simulink model "Katex_FullCar_R2017b_V03"  (R2026a)
settings: Solver=ode1  StopTime=1000  FixedStep=Ts  EnableMultiTasking=on
PostLoadFcn:
  | , if any(exist('dsrtsu_mdlpostloadfcn', 'file') == [2, 3, 6]), try dsrtsu_mdlpostloadfcn('Execute', bdroot); catch fprintf('Error in PostLoadFcn (dsrtsu_mdlpostloadfcn) for model "%s":\n %s\n', bdroot, lasterr); end, end,
  | , if any(exist('dsrtsu_mdlpostloadfcn', 'file') ~= 0), dsrtsu_mdlpostloadfcn('Execute', bdroot); end,
InitFcn:
  | , if any(exist('rtifpga_mdlclblib', 'file') ~= 0), rtifpga_mdlclblib('Init', bdroot); end,
  | 
  | 
  | init
undefined symbols (not defined in the file): locklim_sus, roundN, Ts
libraries: sl_discontinuities x29, simulink_extras x26, simulink x22, mjLib x1
(part 8 of 10)

== system Katex_FullCar_R2017b_V03/DGIST/_Low_Level_Ctrl/Steering_Low_Level_Controller/Torque Mode/Steering Motor Control/Lag compensator(zeta)/a//(s+p) ==
  note: y(n) = [(2-p*Ts)*y(n-1)+a*Ts(u(n)+u(n-1))]/(2+p*Ts)
  note: H(s) = a/(s+p)
  note: s = 2/Ts*(z-1)/(z+1)
  In : Inport
  a : Inport  Port=2
  p : Inport  Port=3
  Constant : Constant  Value=2  SampleTime=Ts
  Product1 : Product  Inputs=*/  RndMeth=Zero
  Product11 : Product  RndMeth=Zero
  Product3 : Product  RndMeth=Zero
  Sum1 : Sum  Inputs=-+  InputSameDT=on  SaturateOnIntegerOverflow=on  OutDataTypeStr=Inherit: Same as first input
  Sum2 : Sum  InputSameDT=on  SaturateOnIntegerOverflow=on  OutDataTypeStr=Inherit: Same as first input
  Sum3 : Sum  InputSameDT=on  SaturateOnIntegerOverflow=on  OutDataTypeStr=Inherit: Same as first input
  Sum4 : Sum  InputSameDT=on  SaturateOnIntegerOverflow=on  OutDataTypeStr=Inherit: Same as first input
  d : UnitDelay  SampleTime=Ts
  d1 : UnitDelay  SampleTime=Ts
  gain : Gain  Gain=Ts  SaturateOnIntegerOverflow=on  OutDataTypeStr=Inherit: Same as input  ParamDataTypeStr=Inherit: Same as input
  gain1 : Gain  Gain=Ts  SaturateOnIntegerOverflow=on  OutDataTypeStr=Inherit: Same as input  ParamDataTypeStr=Inherit: Same as input
  Out : Outport  VectorParamsAs1DForOutWhenUnconnected=off
  wires:
  In/1 -> Sum3/1, d1/1
  d1/1 -> Sum3/2
  Sum3/1 -> gain/1
  Product11/1 -> Sum2/2
  Sum1/1 -> Product11/1
  Constant/1 -> Sum1/2, Sum4/2
  p/1 -> gain1/1
  gain1/1 -> Sum1/1, Sum4/1
  d/1 -> Product11/2
  Sum2/1 -> Product1/1
  Sum4/1 -> Product1/2
  Product1/1 -> Out/1, d/1
  gain/1 -> Product3/1
  a/1 -> Product3/2
  Product3/1 -> Sum2/1

== system Katex_FullCar_R2017b_V03/DGIST/_Low_Level_Ctrl/Steering_Low_Level_Controller/Torque Mode/Steering Motor Control/Poleplacement(PI)1/Integrator1 ==
  note: Integrator
  in : Inport
  "Off : 0 On : 1" : Inport  Port=2
  Divide : Product  Inputs=**
  Sum1 : Sum  InputSameDT=on  SaturateOnIntegerOverflow=on  OutDataTypeStr=Inherit: Same as first input
  Sum2 : Sum  InputSameDT=on  SaturateOnIntegerOverflow=on  OutDataTypeStr=Inherit: Same as first input
  d : UnitDelay  SampleTime=Ts
  d1 : UnitDelay  SampleTime=Ts
  gain : Gain  Gain=Ts/2  SaturateOnIntegerOverflow=on  OutDataTypeStr=Inherit: Same as input  ParamDataTypeStr=Inherit: Same as input
  out : Outport  VectorParamsAs1DForOutWhenUnconnected=off
  wires:
  gain/1 -> Sum2/1
  Sum1/1 -> gain/1
  d1/1 -> Sum1/2
  in/1 -> d1/1, Sum1/1
  Sum2/1 -> Divide/1, out/1
  d/1 -> Sum2/2
  Divide/1 -> d/1
  "Off : 0 On : 1"/1 -> Divide/2

== system Katex_FullCar_R2017b_V03/DGIST/_Low_Level_Ctrl/Steering_Low_Level_Controller/Torque Mode/Steering Motor Control/Steering Ref Mode /If Action Subsystem ==
  In1 : Inport
  Action Port : ActionPort
  Out1 : Outport  VectorParamsAs1DForOutWhenUnconnected=off
  wires:
  In1/1 -> Out1/1

== system Katex_FullCar_R2017b_V03/DGIST/_Low_Level_Ctrl/Steering_Low_Level_Controller/Torque Mode/Steering Motor Control/Steering Ref Mode /If Action Subsystem1 ==
  In1 : Inport
  Action Port : ActionPort
  Out1 : Outport  VectorParamsAs1DForOutWhenUnconnected=off
  wires:
  In1/1 -> Out1/1

== system Katex_FullCar_R2017b_V03/DGIST/_Low_Level_Ctrl/Steering_Low_Level_Controller/Torque Mode/Steering Motor Control/Steering Ref Mode /If Action Subsystem2 ==
  In1 : Inport
  Action Port : ActionPort
  Out1 : Outport  VectorParamsAs1DForOutWhenUnconnected=off
  wires:
  In1/1 -> Out1/1

== system Katex_FullCar_R2017b_V03/DGIST/_Low_Level_Ctrl/Steering_Low_Level_Controller/Torque Mode/Steering Motor Control1/DOB(theta)/Dot ==
  note: Dot
  in : Inport
  Sum1 : Sum  Inputs=+-  InputSameDT=on  SaturateOnIntegerOverflow=on  OutDataTypeStr=Inherit: Same as first input
  Sum2 : Sum  Inputs=+-  InputSameDT=on  SaturateOnIntegerOverflow=on  OutDataTypeStr=Inherit: Same as first input
  d : UnitDelay  SampleTime=Ts
  d1 : UnitDelay  SampleTime=Ts
  gain : Gain  Gain=2/Ts  SaturateOnIntegerOverflow=on  OutDataTypeStr=Inherit: Same as input  ParamDataTypeStr=Inherit: Same as input
  out : Outport  VectorParamsAs1DForOutWhenUnconnected=off
  wires:
  Sum1/1 -> d1/1, out/1
  d1/1 -> Sum1/2
  Sum2/1 -> gain/1
  in/1 -> d/1, Sum2/1
  d/1 -> Sum2/2
  gain/1 -> Sum1/1

== system Katex_FullCar_R2017b_V03/DGIST/_Low_Level_Ctrl/Steering_Low_Level_Controller/Torque Mode/Steering Motor Control1/DOB(theta)/Dot1 ==
  note: Dot
  in : Inport
  Sum1 : Sum  Inputs=+-  InputSameDT=on  SaturateOnIntegerOverflow=on  OutDataTypeStr=Inherit: Same as first input
  Sum2 : Sum  Inputs=+-  InputSameDT=on  SaturateOnIntegerOverflow=on  OutDataTypeStr=Inherit: Same as first input
  d : UnitDelay  SampleTime=Ts
  d1 : UnitDelay  SampleTime=Ts
  gain : Gain  Gain=2/Ts  SaturateOnIntegerOverflow=on  OutDataTypeStr=Inherit: Same as input  ParamDataTypeStr=Inherit: Same as input
  out : Outport  VectorParamsAs1DForOutWhenUnconnected=off
  wires:
  Sum1/1 -> d1/1, out/1
  d1/1 -> Sum1/2
  Sum2/1 -> gain/1
  in/1 -> d/1, Sum2/1
  d/1 -> Sum2/2
  gain/1 -> Sum1/1

== system Katex_FullCar_R2017b_V03/DGIST/_Low_Level_Ctrl/Steering_Low_Level_Controller/Torque Mode/Steering Motor Control1/DOB(theta)/Dot2 ==
  note: Dot
  in : Inport
  Sum1 : Sum  Inputs=+-  InputSameDT=on  SaturateOnIntegerOverflow=on  OutDataTypeStr=Inherit: Same as first input
  Sum2 : Sum  Inputs=+-  InputSameDT=on  SaturateOnIntegerOverflow=on  OutDataTypeStr=Inherit: Same as first input
  d : UnitDelay  SampleTime=Ts
  d1 : UnitDelay  SampleTime=Ts
  gain : Gain  Gain=2/Ts  SaturateOnIntegerOverflow=on  OutDataTypeStr=Inherit: Same as input  ParamDataTypeStr=Inherit: Same as input
  out : Outport  VectorParamsAs1DForOutWhenUnconnected=off
  wires:
  Sum1/1 -> d1/1, out/1
  d1/1 -> Sum1/2
  Sum2/1 -> gain/1
  in/1 -> d/1, Sum2/1
  d/1 -> Sum2/2
  gain/1 -> Sum1/1

== system Katex_FullCar_R2017b_V03/DGIST/_Low_Level_Ctrl/Steering_Low_Level_Controller/Torque Mode/Steering Motor Control1/DOB(theta)/Second order LPF ==
  note: y(n) = [Ts^2*w^2*{x(n)+2*x(n-1)+x(n-2)}-(2*w^2*Ts^2-8)*y(n-1)-(4+w^2*Ts^2+2*zeta*Ts*w)*y(n-2)]
      | /(4+w^2*Ts^2+2*zeta*Ts*w)
  note: H(s) = w^2/(s^2+2*zeta*w*s+w^2)
  note: s = 2/Ts*(z-1)/(z+1)
  In : Inport
  fc : Inport  Port=2
  zeta : Inport  Port=3
  Constant : Constant  Value=Ts  SampleTime=Ts
  Constant1 : Constant  Value=8  SampleTime=Ts
  Constant2 : Constant  Value=4  SampleTime=Ts
  Delay : Delay  InitialCondition=0  SampleTime=Ts
  Delay1 : Delay  DelayLength=1  InitialCondition=0  SampleTime=Ts
  Delay2 : Delay  DelayLength=1  InitialCondition=0  SampleTime=Ts
  Delay3 : Delay  InitialCondition=0  SampleTime=Ts
  Product1 : Product  Inputs=*/  RndMeth=Zero
  Product2 : Product  Inputs=4  RndMeth=Zero
  Product3 : Product  RndMeth=Zero
  Product4 : Product  RndMeth=Zero
  Sum1 : Sum  Inputs=+-  InputSameDT=on  SaturateOnIntegerOverflow=on  OutDataTypeStr=Inherit: Same as first input
  Sum2 : Sum  Inputs=+-  InputSameDT=on  SaturateOnIntegerOverflow=on  OutDataTypeStr=Inherit: Same as first input
  Sum3 : Sum  Inputs=+++  InputSameDT=on  SaturateOnIntegerOverflow=on  OutDataTypeStr=Inherit: Same as first input
  Sum4 : Sum  Inputs=+-  InputSameDT=on  SaturateOnIntegerOverflow=on  OutDataTypeStr=Inherit: Same as first input
  Sum5 : Sum  Inputs=+-+  InputSameDT=on  SaturateOnIntegerOverflow=on  OutDataTypeStr=Inherit: Same as first input
  Sum6 : Sum  Inputs=+++  InputSameDT=on  SaturateOnIntegerOverflow=on  OutDataTypeStr=Inherit: Same as first input
  gain1 : Gain  Gain=2  SaturateOnIntegerOverflow=on  OutDataTypeStr=Inherit: Same as input  ParamDataTypeStr=Inherit: Same as input
  gain2 : Gain  Gain=2*pi  SaturateOnIntegerOverflow=on  OutDataTypeStr=Inherit: Same as input  ParamDataTypeStr=Inherit: Same as input
  gain3 : Gain  Gain=2  SaturateOnIntegerOverflow=on  OutDataTypeStr=Inherit: Same as input  ParamDataTypeStr=Inherit: Same as input
  gain4 : Gain  Gain=4  SaturateOnIntegerOverflow=on  OutDataTypeStr=Inherit: Same as input  ParamDataTypeStr=Inherit: Same as input
  "x(n), x(n-1), x(n-2)" : Product  RndMeth=Zero
  y(n-1) : Product  RndMeth=Zero
  y(n-2) : Product  RndMeth=Zero
  Dist_hat : Outport  VectorParamsAs1DForOutWhenUnconnected=off
  wires:
  Product1/1 -> Dist_hat/1, Delay3/1, Delay2/1
  Sum2/1 -> Product1/1
  fc/1 -> gain2/1
  In/1 -> Delay1/1, Delay/1, Sum3/1
  gain2/1 -> Product3/1, Product2/2, Product2/1
  Constant/1 -> Product3/2, Product2/4, Product2/3
  Delay1/1 -> gain1/1
  gain1/1 -> Sum3/2
  Delay/1 -> Sum3/3
  Sum3/1 -> "x(n), x(n-1), x(n-2)"/1
  Product2/1 -> Sum5/1, Sum6/1, "x(n), x(n-1), x(n-2)"/2, gain3/1
  "x(n), x(n-1), x(n-2)"/1 -> Sum1/1
  Sum1/1 -> Sum2/1
  y(n-1)/1 -> Sum1/2
  Sum4/1 -> y(n-1)/1
  gain3/1 -> Sum4/1
  Constant1/1 -> Sum4/2
  Delay2/1 -> y(n-1)/2
  Product3/1 -> gain4/1
  Constant2/1 -> Sum5/3, Sum6/3
  Sum5/1 -> y(n-2)/1
  Delay3/1 -> y(n-2)/2
  y(n-2)/1 -> Sum2/2
  Sum6/1 -> Product1/2
  zeta/1 -> Product4/2
  gain4/1 -> Product4/1
  Product4/1 -> Sum6/2, Sum5/2

== system Katex_FullCar_R2017b_V03/DGIST/_Low_Level_Ctrl/Steering_Low_Level_Controller/Torque Mode/Steering Motor Control1/Feedforward(theta)/Dot ==
  note: Dot
  in : Inport
  Sum1 : Sum  Inputs=+-  InputSameDT=on  SaturateOnIntegerOverflow=on  OutDataTypeStr=Inherit: Same as first input
  Sum2 : Sum  Inputs=+-  InputSameDT=on  SaturateOnIntegerOverflow=on  OutDataTypeStr=Inherit: Same as first input
  d : UnitDelay  SampleTime=Ts
  d1 : UnitDelay  SampleTime=Ts
  gain : Gain  Gain=2/Ts  SaturateOnIntegerOverflow=on  OutDataTypeStr=Inherit: Same as input  ParamDataTypeStr=Inherit: Same as input
  out : Outport  VectorParamsAs1DForOutWhenUnconnected=off
  wires:
  Sum1/1 -> d1/1, out/1
  d1/1 -> Sum1/2
  Sum2/1 -> gain/1
  in/1 -> d/1, Sum2/1
  d/1 -> Sum2/2
  gain/1 -> Sum1/1

== system Katex_FullCar_R2017b_V03/DGIST/_Low_Level_Ctrl/Steering_Low_Level_Controller/Torque Mode/Steering Motor Control1/Feedforward(theta)/Dot1 ==
  note: Dot
  in : Inport
  Sum1 : Sum  Inputs=+-  InputSameDT=on  SaturateOnIntegerOverflow=on  OutDataTypeStr=Inherit: Same as first input
  Sum2 : Sum  Inputs=+-  InputSameDT=on  SaturateOnIntegerOverflow=on  OutDataTypeStr=Inherit: Same as first input
  d : UnitDelay  SampleTime=Ts
  d1 : UnitDelay  SampleTime=Ts
  gain : Gain  Gain=2/Ts  SaturateOnIntegerOverflow=on  OutDataTypeStr=Inherit: Same as input  ParamDataTypeStr=Inherit: Same as input
  out : Outport  VectorParamsAs1DForOutWhenUnconnected=off
  wires:
  Sum1/1 -> d1/1, out/1
  d1/1 -> Sum1/2
  Sum2/1 -> gain/1
  in/1 -> d/1, Sum2/1
  d/1 -> Sum2/2
  gain/1 -> Sum1/1

== system Katex_FullCar_R2017b_V03/DGIST/_Low_Level_Ctrl/Steering_Low_Level_Controller/Torque Mode/Steering Motor Control1/Feedforward(theta)/Dot2 ==
  note: Dot
  in : Inport
  Sum1 : Sum  Inputs=+-  InputSameDT=on  SaturateOnIntegerOverflow=on  OutDataTypeStr=Inherit: Same as first input
  Sum2 : Sum  Inputs=+-  InputSameDT=on  SaturateOnIntegerOverflow=on  OutDataTypeStr=Inherit: Same as first input
  d : UnitDelay  SampleTime=Ts
  d1 : UnitDelay  SampleTime=Ts
  gain : Gain  Gain=2/Ts  SaturateOnIntegerOverflow=on  OutDataTypeStr=Inherit: Same as input  ParamDataTypeStr=Inherit: Same as input
  out : Outport  VectorParamsAs1DForOutWhenUnconnected=off
  wires:
  Sum1/1 -> d1/1, out/1
  d1/1 -> Sum1/2
  Sum2/1 -> gain/1
  in/1 -> d/1, Sum2/1
  d/1 -> Sum2/2
  gain/1 -> Sum1/1

== system Katex_FullCar_R2017b_V03/DGIST/_Low_Level_Ctrl/Steering_Low_Level_Controller/Torque Mode/Steering Motor Control1/Feedforward(theta)/Second order LPF ==
  note: y(n) = [Ts^2*w^2*{x(n)+2*x(n-1)+x(n-2)}-(2*w^2*Ts^2-8)*y(n-1)-(4+w^2*Ts^2+2*zeta*Ts*w)*y(n-2)]
      | /(4+w^2*Ts^2+2*zeta*Ts*w)
  note: H(s) = w^2/(s^2+2*zeta*w*s+w^2)
  note: s = 2/Ts*(z-1)/(z+1)
  In : Inport
  fc : Inport  Port=2
  zeta : Inport  Port=3
  Constant : Constant  Value=Ts  SampleTime=Ts
  Constant1 : Constant  Value=8  SampleTime=Ts
  Constant2 : Constant  Value=4  SampleTime=Ts
  Delay : Delay  InitialCondition=0  SampleTime=Ts
  Delay1 : Delay  DelayLength=1  InitialCondition=0  SampleTime=Ts
  Delay2 : Delay  DelayLength=1  InitialCondition=0  SampleTime=Ts
  Delay3 : Delay  InitialCondition=0  SampleTime=Ts
  Product1 : Product  Inputs=*/  RndMeth=Zero
  Product2 : Product  Inputs=4  RndMeth=Zero
  Product3 : Product  RndMeth=Zero
  Product4 : Product  RndMeth=Zero
  Sum1 : Sum  Inputs=+-  InputSameDT=on  SaturateOnIntegerOverflow=on  OutDataTypeStr=Inherit: Same as first input
  Sum2 : Sum  Inputs=+-  InputSameDT=on  SaturateOnIntegerOverflow=on  OutDataTypeStr=Inherit: Same as first input
  Sum3 : Sum  Inputs=+++  InputSameDT=on  SaturateOnIntegerOverflow=on  OutDataTypeStr=Inherit: Same as first input
  Sum4 : Sum  Inputs=+-  InputSameDT=on  SaturateOnIntegerOverflow=on  OutDataTypeStr=Inherit: Same as first input
  Sum5 : Sum  Inputs=+-+  InputSameDT=on  SaturateOnIntegerOverflow=on  OutDataTypeStr=Inherit: Same as first input
  Sum6 : Sum  Inputs=+++  InputSameDT=on  SaturateOnIntegerOverflow=on  OutDataTypeStr=Inherit: Same as first input
  gain1 : Gain  Gain=2  SaturateOnIntegerOverflow=on  OutDataTypeStr=Inherit: Same as input  ParamDataTypeStr=Inherit: Same as input
  gain2 : Gain  Gain=2*pi  SaturateOnIntegerOverflow=on  OutDataTypeStr=Inherit: Same as input  ParamDataTypeStr=Inherit: Same as input
  gain3 : Gain  Gain=2  SaturateOnIntegerOverflow=on  OutDataTypeStr=Inherit: Same as input  ParamDataTypeStr=Inherit: Same as input
  gain4 : Gain  Gain=4  SaturateOnIntegerOverflow=on  OutDataTypeStr=Inherit: Same as input  ParamDataTypeStr=Inherit: Same as input
  "x(n), x(n-1), x(n-2)" : Product  RndMeth=Zero
  y(n-1) : Product  RndMeth=Zero
  y(n-2) : Product  RndMeth=Zero
  Out : Outport  VectorParamsAs1DForOutWhenUnconnected=off
  wires:
  Product1/1 -> Out/1, Delay3/1, Delay2/1
  Sum2/1 -> Product1/1
  fc/1 -> gain2/1
  In/1 -> Delay1/1, Delay/1, Sum3/1
  gain2/1 -> Product3/1, Product2/2, Product2/1
  Constant/1 -> Product3/2, Product2/4, Product2/3
  Delay1/1 -> gain1/1
  gain1/1 -> Sum3/2
  Delay/1 -> Sum3/3
  Sum3/1 -> "x(n), x(n-1), x(n-2)"/1
  Product2/1 -> Sum5/1, Sum6/1, "x(n), x(n-1), x(n-2)"/2, gain3/1
  "x(n), x(n-1), x(n-2)"/1 -> Sum1/1
  Sum1/1 -> Sum2/1
  y(n-1)/1 -> Sum1/2
  Sum4/1 -> y(n-1)/1
  gain3/1 -> Sum4/1
  Constant1/1 -> Sum4/2
  Delay2/1 -> y(n-1)/2
  Product3/1 -> gain4/1
  Constant2/1 -> Sum5/3, Sum6/3
  Sum5/1 -> y(n-2)/1
  Delay3/1 -> y(n-2)/2
  y(n-2)/1 -> Sum2/2
  Sum6/1 -> Product1/2
  zeta/1 -> Product4/2
  gain4/1 -> Product4/1
  Product4/1 -> Sum6/2, Sum5/2

== system Katex_FullCar_R2017b_V03/DGIST/_Low_Level_Ctrl/Steering_Low_Level_Controller/Torque Mode/Steering Motor Control1/Lag compensator(zeta)/Dot1 ==
  note: Dot
  in : Inport
  Sum1 : Sum  Inputs=+-  InputSameDT=on  SaturateOnIntegerOverflow=on  OutDataTypeStr=Inherit: Same as first input
  Sum2 : Sum  Inputs=+-  InputSameDT=on  SaturateOnIntegerOverflow=on  OutDataTypeStr=Inherit: Same as first input
  d : UnitDelay  SampleTime=Ts
  d1 : UnitDelay  SampleTime=Ts
  gain : Gain  Gain=2/Ts  SaturateOnIntegerOverflow=on  OutDataTypeStr=Inherit: Same as input  ParamDataTypeStr=Inherit: Same as input
  out : Outport  VectorParamsAs1DForOutWhenUnconnected=off
  wires:
  Sum1/1 -> d1/1, out/1
  d1/1 -> Sum1/2
  Sum2/1 -> gain/1
  in/1 -> d/1, Sum2/1
  d/1 -> Sum2/2
  gain/1 -> Sum1/1

== system Katex_FullCar_R2017b_V03/DGIST/_Low_Level_Ctrl/Steering_Low_Level_Controller/Torque Mode/Steering Motor Control1/Lag compensator(zeta)/a//(s+p) ==
  note: y(n) = [(2-p*Ts)*y(n-1)+a*Ts(u(n)+u(n-1))]/(2+p*Ts)
  note: H(s) = a/(s+p)
  note: s = 2/Ts*(z-1)/(z+1)
  In : Inport
  a : Inport  Port=2
  p : Inport  Port=3
  Constant : Constant  Value=2  SampleTime=Ts
  Product1 : Product  Inputs=*/  RndMeth=Zero
  Product11 : Product  RndMeth=Zero
  Product3 : Product  RndMeth=Zero
  Sum1 : Sum  Inputs=-+  InputSameDT=on  SaturateOnIntegerOverflow=on  OutDataTypeStr=Inherit: Same as first input
  Sum2 : Sum  InputSameDT=on  SaturateOnIntegerOverflow=on  OutDataTypeStr=Inherit: Same as first input
  Sum3 : Sum  InputSameDT=on  SaturateOnIntegerOverflow=on  OutDataTypeStr=Inherit: Same as first input
  Sum4 : Sum  InputSameDT=on  SaturateOnIntegerOverflow=on  OutDataTypeStr=Inherit: Same as first input
  d : UnitDelay  SampleTime=Ts
  d1 : UnitDelay  SampleTime=Ts
  gain : Gain  Gain=Ts  SaturateOnIntegerOverflow=on  OutDataTypeStr=Inherit: Same as input  ParamDataTypeStr=Inherit: Same as input
  gain1 : Gain  Gain=Ts  SaturateOnIntegerOverflow=on  OutDataTypeStr=Inherit: Same as input  ParamDataTypeStr=Inherit: Same as input
  Out : Outport  VectorParamsAs1DForOutWhenUnconnected=off
  wires:
  In/1 -> Sum3/1, d1/1
  d1/1 -> Sum3/2
  Sum3/1 -> gain/1
  Product11/1 -> Sum2/2
  Sum1/1 -> Product11/1
  Constant/1 -> Sum1/2, Sum4/2
  p/1 -> gain1/1
  gain1/1 -> Sum1/1, Sum4/1
  d/1 -> Product11/2
  Sum2/1 -> Product1/1
  Sum4/1 -> Product1/2
  Product1/1 -> Out/1, d/1
  gain/1 -> Product3/1
  a/1 -> Product3/2
  Product3/1 -> Sum2/1

== system Katex_FullCar_R2017b_V03/DGIST/_Low_Level_Ctrl/Steering_Low_Level_Controller/Torque Mode/Steering Motor Control2/DOB(omega)/Dot2 ==
  note: Dot
  in : Inport
  Sum1 : Sum  Inputs=+-  InputSameDT=on  SaturateOnIntegerOverflow=on  OutDataTypeStr=Inherit: Same as first input
  Sum2 : Sum  Inputs=+-  InputSameDT=on  SaturateOnIntegerOverflow=on  OutDataTypeStr=Inherit: Same as first input
  d : UnitDelay  SampleTime=Ts
  d1 : UnitDelay  SampleTime=Ts
  gain : Gain  Gain=2/Ts  SaturateOnIntegerOverflow=on  OutDataTypeStr=Inherit: Same as input  ParamDataTypeStr=Inherit: Same as input
  out : Outport  VectorParamsAs1DForOutWhenUnconnected=off
  wires:
  Sum1/1 -> d1/1, out/1
  d1/1 -> Sum1/2
  Sum2/1 -> gain/1
  in/1 -> d/1, Sum2/1
  d/1 -> Sum2/2
  gain/1 -> Sum1/1

== system Katex_FullCar_R2017b_V03/DGIST/_Low_Level_Ctrl/Steering_Low_Level_Controller/Torque Mode/Steering Motor Control2/DOB(omega)/LPF ==
  note: LPF : tau = 1/(2*pi*fc)
  note: y(n) = [Ts*{x(n)+x(n-1)}+(2*tau-Ts)*y(n-1)]/(2*tau+Ts)
  note: H(s) = 1/(tau*s+1)
  note: s = 2/Ts*(z-1)/(z+1)
  In : Inport
  fc : Inport  Port=2
  Constant : Constant  Value=Ts  SampleTime=Ts
  Constant1 : Constant  SampleTime=Ts
  Product1 : Product  Inputs=*/  RndMeth=Zero
  Product11 : Product  RndMeth=Zero
  Product2 : Product  Inputs=*/  RndMeth=Zero
  Sum1 : Sum  Inputs=+-  InputSameDT=on  SaturateOnIntegerOverflow=on  OutDataTypeStr=Inherit: Same as first input
  Sum2 : Sum  InputSameDT=on  SaturateOnIntegerOverflow=on  OutDataTypeStr=Inherit: Same as first input
  Sum3 : Sum  InputSameDT=on  SaturateOnIntegerOverflow=on  OutDataTypeStr=Inherit: Same as first input
  Sum4 : Sum  InputSameDT=on  SaturateOnIntegerOverflow=on  OutDataTypeStr=Inherit: Same as first input
  d : UnitDelay  SampleTime=Ts
  d1 : UnitDelay  SampleTime=Ts
  gain : Gain  Gain=Ts  SaturateOnIntegerOverflow=on  OutDataTypeStr=Inherit: Same as input  ParamDataTypeStr=Inherit: Same as input
  gain1 : Gain  Gain=2  SaturateOnIntegerOverflow=on  OutDataTypeStr=Inherit: Same as input  ParamDataTypeStr=Inherit: Same as input
  gain2 : Gain  Gain=2*pi  SaturateOnIntegerOverflow=on  OutDataTypeStr=Inherit: Same as input  ParamDataTypeStr=Inherit: Same as input
  Out : Outport  VectorParamsAs1DForOutWhenUnconnected=off
  wires:
  In/1 -> Sum3/1, d1/1
  d1/1 -> Sum3/2
  Sum3/1 -> gain/1
  gain/1 -> Sum2/1
  Product11/1 -> Sum2/2
  Sum1/1 -> Product11/1
  Constant/1 -> Sum1/2, Sum4/2
  fc/1 -> gain2/1
  gain1/1 -> Sum1/1, Sum4/1
  d/1 -> Product11/2
  Sum2/1 -> Product1/1
  Sum4/1 -> Product1/2
  Product1/1 -> Out/1, d/1
  Product2/1 -> gain1/1
  Constant1/1 -> Product2/1
  gain2/1 -> Product2/2

== system Katex_FullCar_R2017b_V03/DGIST/_Low_Level_Ctrl/Steering_Low_Level_Controller/Torque Mode/Steering Motor Control2/DOB(theta)/Dot ==
  note: Dot
  in : Inport
  Sum1 : Sum  Inputs=+-  InputSameDT=on  SaturateOnIntegerOverflow=on  OutDataTypeStr=Inherit: Same as first input
  Sum2 : Sum  Inputs=+-  InputSameDT=on  SaturateOnIntegerOverflow=on  OutDataTypeStr=Inherit: Same as first input
  d : UnitDelay  SampleTime=Ts
  d1 : UnitDelay  SampleTime=Ts
  gain : Gain  Gain=2/Ts  SaturateOnIntegerOverflow=on  OutDataTypeStr=Inherit: Same as input  ParamDataTypeStr=Inherit: Same as input
  out : Outport  VectorParamsAs1DForOutWhenUnconnected=off
  wires:
  Sum1/1 -> d1/1, out/1
  d1/1 -> Sum1/2
  Sum2/1 -> gain/1
  in/1 -> d/1, Sum2/1
  d/1 -> Sum2/2
  gain/1 -> Sum1/1

== system Katex_FullCar_R2017b_V03/DGIST/_Low_Level_Ctrl/Steering_Low_Level_Controller/Torque Mode/Steering Motor Control2/DOB(theta)/Dot1 ==
  note: Dot
  in : Inport
  Sum1 : Sum  Inputs=+-  InputSameDT=on  SaturateOnIntegerOverflow=on  OutDataTypeStr=Inherit: Same as first input
  Sum2 : Sum  Inputs=+-  InputSameDT=on  SaturateOnIntegerOverflow=on  OutDataTypeStr=Inherit: Same as first input
  d : UnitDelay  SampleTime=Ts
  d1 : UnitDelay  SampleTime=Ts
  gain : Gain  Gain=2/Ts  SaturateOnIntegerOverflow=on  OutDataTypeStr=Inherit: Same as input  ParamDataTypeStr=Inherit: Same as input
  out : Outport  VectorParamsAs1DForOutWhenUnconnected=off
  wires:
  Sum1/1 -> d1/1, out/1
  d1/1 -> Sum1/2
  Sum2/1 -> gain/1
  in/1 -> d/1, Sum2/1
  d/1 -> Sum2/2
  gain/1 -> Sum1/1

== system Katex_FullCar_R2017b_V03/DGIST/_Low_Level_Ctrl/Steering_Low_Level_Controller/Torque Mode/Steering Motor Control2/DOB(theta)/Dot2 ==
  note: Dot
  in : Inport
  Sum1 : Sum  Inputs=+-  InputSameDT=on  SaturateOnIntegerOverflow=on  OutDataTypeStr=Inherit: Same as first input
  Sum2 : Sum  Inputs=+-  InputSameDT=on  SaturateOnIntegerOverflow=on  OutDataTypeStr=Inherit: Same as first input
  d : UnitDelay  SampleTime=Ts
  d1 : UnitDelay  SampleTime=Ts
  gain : Gain  Gain=2/Ts  SaturateOnIntegerOverflow=on  OutDataTypeStr=Inherit: Same as input  ParamDataTypeStr=Inherit: Same as input
  out : Outport  VectorParamsAs1DForOutWhenUnconnected=off
  wires:
  Sum1/1 -> d1/1, out/1
  d1/1 -> Sum1/2
  Sum2/1 -> gain/1
  in/1 -> d/1, Sum2/1
  d/1 -> Sum2/2
  gain/1 -> Sum1/1

== system Katex_FullCar_R2017b_V03/DGIST/_Low_Level_Ctrl/Steering_Low_Level_Controller/Torque Mode/Steering Motor Control2/DOB(theta)/Second order LPF ==
  note: y(n) = [Ts^2*w^2*{x(n)+2*x(n-1)+x(n-2)}-(2*w^2*Ts^2-8)*y(n-1)-(4+w^2*Ts^2+2*zeta*Ts*w)*y(n-2)]
      | /(4+w^2*Ts^2+2*zeta*Ts*w)
  note: H(s) = w^2/(s^2+2*zeta*w*s+w^2)
  note: s = 2/Ts*(z-1)/(z+1)
  In : Inport
  fc : Inport  Port=2
  zeta : Inport  Port=3
  Constant : Constant  Value=Ts  SampleTime=Ts
  Constant1 : Constant  Value=8  SampleTime=Ts
  Constant2 : Constant  Value=4  SampleTime=Ts
  Delay : Delay  InitialCondition=0  SampleTime=Ts
  Delay1 : Delay  DelayLength=1  InitialCondition=0  SampleTime=Ts
  Delay2 : Delay  DelayLength=1  InitialCondition=0  SampleTime=Ts
  Delay3 : Delay  InitialCondition=0  SampleTime=Ts
  Product1 : Product  Inputs=*/  RndMeth=Zero
  Product2 : Product  Inputs=4  RndMeth=Zero
  Product3 : Product  RndMeth=Zero
  Product4 : Product  RndMeth=Zero
  Sum1 : Sum  Inputs=+-  InputSameDT=on  SaturateOnIntegerOverflow=on  OutDataTypeStr=Inherit: Same as first input
  Sum2 : Sum  Inputs=+-  InputSameDT=on  SaturateOnIntegerOverflow=on  OutDataTypeStr=Inherit: Same as first input
  Sum3 : Sum  Inputs=+++  InputSameDT=on  SaturateOnIntegerOverflow=on  OutDataTypeStr=Inherit: Same as first input
  Sum4 : Sum  Inputs=+-  InputSameDT=on  SaturateOnIntegerOverflow=on  OutDataTypeStr=Inherit: Same as first input
  Sum5 : Sum  Inputs=+-+  InputSameDT=on  SaturateOnIntegerOverflow=on  OutDataTypeStr=Inherit: Same as first input
  Sum6 : Sum  Inputs=+++  InputSameDT=on  SaturateOnIntegerOverflow=on  OutDataTypeStr=Inherit: Same as first input
  gain1 : Gain  Gain=2  SaturateOnIntegerOverflow=on  OutDataTypeStr=Inherit: Same as input  ParamDataTypeStr=Inherit: Same as input
  gain2 : Gain  Gain=2*pi  SaturateOnIntegerOverflow=on  OutDataTypeStr=Inherit: Same as input  ParamDataTypeStr=Inherit: Same as input
  gain3 : Gain  Gain=2  SaturateOnIntegerOverflow=on  OutDataTypeStr=Inherit: Same as input  ParamDataTypeStr=Inherit: Same as input
  gain4 : Gain  Gain=4  SaturateOnIntegerOverflow=on  OutDataTypeStr=Inherit: Same as input  ParamDataTypeStr=Inherit: Same as input
  "x(n), x(n-1), x(n-2)" : Product  RndMeth=Zero
  y(n-1) : Product  RndMeth=Zero
  y(n-2) : Product  RndMeth=Zero
  Dist_hat : Outport  VectorParamsAs1DForOutWhenUnconnected=off
  wires:
  Product1/1 -> Dist_hat/1, Delay3/1, Delay2/1
  Sum2/1 -> Product1/1
  fc/1 -> gain2/1
  In/1 -> Delay1/1, Delay/1, Sum3/1
  gain2/1 -> Product3/1, Product2/2, Product2/1
  Constant/1 -> Product3/2, Product2/4, Product2/3
  Delay1/1 -> gain1/1
  gain1/1 -> Sum3/2
  Delay/1 -> Sum3/3
  Sum3/1 -> "x(n), x(n-1), x(n-2)"/1
  Product2/1 -> Sum5/1, Sum6/1, "x(n), x(n-1), x(n-2)"/2, gain3/1
  "x(n), x(n-1), x(n-2)"/1 -> Sum1/1
  Sum1/1 -> Sum2/1
  y(n-1)/1 -> Sum1/2
  Sum4/1 -> y(n-1)/1
  gain3/1 -> Sum4/1
  Constant1/1 -> Sum4/2
  Delay2/1 -> y(n-1)/2
  Product3/1 -> gain4/1
  Constant2/1 -> Sum5/3, Sum6/3
  Sum5/1 -> y(n-2)/1
  Delay3/1 -> y(n-2)/2
  y(n-2)/1 -> Sum2/2
  Sum6/1 -> Product1/2
  zeta/1 -> Product4/2
  gain4/1 -> Product4/1
  Product4/1 -> Sum6/2, Sum5/2

== system Katex_FullCar_R2017b_V03/DGIST/_Low_Level_Ctrl/Steering_Low_Level_Controller/Torque Mode/Steering Motor Control2/Feedforward(omega)/Dot2 ==
  note: Dot
  in : Inport
  Sum1 : Sum  Inputs=+-  InputSameDT=on  SaturateOnIntegerOverflow=on  OutDataTypeStr=Inherit: Same as first input
  Sum2 : Sum  Inputs=+-  InputSameDT=on  SaturateOnIntegerOverflow=on  OutDataTypeStr=Inherit: Same as first input
  d : UnitDelay  SampleTime=Ts
  d1 : UnitDelay  SampleTime=Ts
  gain : Gain  Gain=2/Ts  SaturateOnIntegerOverflow=on  OutDataTypeStr=Inherit: Same as input  ParamDataTypeStr=Inherit: Same as input
  out : Outport  VectorParamsAs1DForOutWhenUnconnected=off
  wires:
  Sum1/1 -> d1/1, out/1
  d1/1 -> Sum1/2
  Sum2/1 -> gain/1
  in/1 -> d/1, Sum2/1
  d/1 -> Sum2/2
  gain/1 -> Sum1/1

== system Katex_FullCar_R2017b_V03/DGIST/_Low_Level_Ctrl/Steering_Low_Level_Controller/Torque Mode/Steering Motor Control2/Feedforward(omega)/LPF ==
  note: LPF : tau = 1/(2*pi*fc)
  note: y(n) = [Ts*{x(n)+x(n-1)}+(2*tau-Ts)*y(n-1)]/(2*tau+Ts)
  note: H(s) = 1/(tau*s+1)
  note: s = 2/Ts*(z-1)/(z+1)
  In : Inport
  fc : Inport  Port=2
  Constant : Constant  Value=Ts  SampleTime=Ts
  Constant1 : Constant  SampleTime=Ts
  Product1 : Product  Inputs=*/  RndMeth=Zero
  Product11 : Product  RndMeth=Zero
  Product2 : Product  Inputs=*/  RndMeth=Zero
  Sum1 : Sum  Inputs=+-  InputSameDT=on  SaturateOnIntegerOverflow=on  OutDataTypeStr=Inherit: Same as first input
  Sum2 : Sum  InputSameDT=on  SaturateOnIntegerOverflow=on  OutDataTypeStr=Inherit: Same as first input
  Sum3 : Sum  InputSameDT=on  SaturateOnIntegerOverflow=on  OutDataTypeStr=Inherit: Same as first input
  Sum4 : Sum  InputSameDT=on  SaturateOnIntegerOverflow=on  OutDataTypeStr=Inherit: Same as first input
  d : UnitDelay  SampleTime=Ts
  d1 : UnitDelay  SampleTime=Ts
  gain : Gain  Gain=Ts  SaturateOnIntegerOverflow=on  OutDataTypeStr=Inherit: Same as input  ParamDataTypeStr=Inherit: Same as input
  gain1 : Gain  Gain=2  SaturateOnIntegerOverflow=on  OutDataTypeStr=Inherit: Same as input  ParamDataTypeStr=Inherit: Same as input
  gain2 : Gain  Gain=2*pi  SaturateOnIntegerOverflow=on  OutDataTypeStr=Inherit: Same as input  ParamDataTypeStr=Inherit: Same as input
  Out : Outport  VectorParamsAs1DForOutWhenUnconnected=off
  wires:
  In/1 -> Sum3/1, d1/1
  d1/1 -> Sum3/2
  Sum3/1 -> gain/1
  gain/1 -> Sum2/1
  Product11/1 -> Sum2/2
  Sum1/1 -> Product11/1
  Constant/1 -> Sum1/2, Sum4/2
  fc/1 -> gain2/1
  gain1/1 -> Sum1/1, Sum4/1
  d/1 -> Product11/2
  Sum2/1 -> Product1/1
  Sum4/1 -> Product1/2
  Product1/1 -> Out/1, d/1
  Product2/1 -> gain1/1
  Constant1/1 -> Product2/1
  gain2/1 -> Product2/2

== system Katex_FullCar_R2017b_V03/DGIST/_Low_Level_Ctrl/Steering_Low_Level_Controller/Torque Mode/Steering Motor Control2/Feedforward(theta)/Dot ==
  note: Dot
  in : Inport
  Sum1 : Sum  Inputs=+-  InputSameDT=on  SaturateOnIntegerOverflow=on  OutDataTypeStr=Inherit: Same as first input
  Sum2 : Sum  Inputs=+-  InputSameDT=on  SaturateOnIntegerOverflow=on  OutDataTypeStr=Inherit: Same as first input
  d : UnitDelay  SampleTime=Ts
  d1 : UnitDelay  SampleTime=Ts
  gain : Gain  Gain=2/Ts  SaturateOnIntegerOverflow=on  OutDataTypeStr=Inherit: Same as input  ParamDataTypeStr=Inherit: Same as input
  out : Outport  VectorParamsAs1DForOutWhenUnconnected=off
  wires:
  Sum1/1 -> d1/1, out/1
  d1/1 -> Sum1/2
  Sum2/1 -> gain/1
  in/1 -> d/1, Sum2/1
  d/1 -> Sum2/2
  gain/1 -> Sum1/1

== system Katex_FullCar_R2017b_V03/DGIST/_Low_Level_Ctrl/Steering_Low_Level_Controller/Torque Mode/Steering Motor Control2/Feedforward(theta)/Dot1 ==
  note: Dot
  in : Inport
  Sum1 : Sum  Inputs=+-  InputSameDT=on  SaturateOnIntegerOverflow=on  OutDataTypeStr=Inherit: Same as first input
  Sum2 : Sum  Inputs=+-  InputSameDT=on  SaturateOnIntegerOverflow=on  OutDataTypeStr=Inherit: Same as first input
  d : UnitDelay  SampleTime=Ts
  d1 : UnitDelay  SampleTime=Ts
  gain : Gain  Gain=2/Ts  SaturateOnIntegerOverflow=on  OutDataTypeStr=Inherit: Same as input  ParamDataTypeStr=Inherit: Same as input
  out : Outport  VectorParamsAs1DForOutWhenUnconnected=off
  wires:
  Sum1/1 -> d1/1, out/1
  d1/1 -> Sum1/2
  Sum2/1 -> gain/1
  in/1 -> d/1, Sum2/1
  d/1 -> Sum2/2
  gain/1 -> Sum1/1

== system Katex_FullCar_R2017b_V03/DGIST/_Low_Level_Ctrl/Steering_Low_Level_Controller/Torque Mode/Steering Motor Control2/Feedforward(theta)/Dot2 ==
  note: Dot
  in : Inport
  Sum1 : Sum  Inputs=+-  InputSameDT=on  SaturateOnIntegerOverflow=on  OutDataTypeStr=Inherit: Same as first input
  Sum2 : Sum  Inputs=+-  InputSameDT=on  SaturateOnIntegerOverflow=on  OutDataTypeStr=Inherit: Same as first input
  d : UnitDelay  SampleTime=Ts
  d1 : UnitDelay  SampleTime=Ts
  gain : Gain  Gain=2/Ts  SaturateOnIntegerOverflow=on  OutDataTypeStr=Inherit: Same as input  ParamDataTypeStr=Inherit: Same as input
  out : Outport  VectorParamsAs1DForOutWhenUnconnected=off
  wires:
  Sum1/1 -> d1/1, out/1
  d1/1 -> Sum1/2
  Sum2/1 -> gain/1
  in/1 -> d/1, Sum2/1
  d/1 -> Sum2/2
  gain/1 -> Sum1/1

== system Katex_FullCar_R2017b_V03/DGIST/_Low_Level_Ctrl/Steering_Low_Level_Controller/Torque Mode/Steering Motor Control2/Feedforward(theta)/Second order LPF ==
  note: y(n) = [Ts^2*w^2*{x(n)+2*x(n-1)+x(n-2)}-(2*w^2*Ts^2-8)*y(n-1)-(4+w^2*Ts^2+2*zeta*Ts*w)*y(n-2)]
      | /(4+w^2*Ts^2+2*zeta*Ts*w)
  note: H(s) = w^2/(s^2+2*zeta*w*s+w^2)
  note: s = 2/Ts*(z-1)/(z+1)
  In : Inport
  fc : Inport  Port=2
  zeta : Inport  Port=3
  Constant : Constant  Value=Ts  SampleTime=Ts
  Constant1 : Constant  Value=8  SampleTime=Ts
  Constant2 : Constant  Value=4  SampleTime=Ts
  Delay : Delay  InitialCondition=0  SampleTime=Ts
  Delay1 : Delay  DelayLength=1  InitialCondition=0  SampleTime=Ts
  Delay2 : Delay  DelayLength=1  InitialCondition=0  SampleTime=Ts
  Delay3 : Delay  InitialCondition=0  SampleTime=Ts
  Product1 : Product  Inputs=*/  RndMeth=Zero
  Product2 : Product  Inputs=4  RndMeth=Zero
  Product3 : Product  RndMeth=Zero
  Product4 : Product  RndMeth=Zero
  Sum1 : Sum  Inputs=+-  InputSameDT=on  SaturateOnIntegerOverflow=on  OutDataTypeStr=Inherit: Same as first input
  Sum2 : Sum  Inputs=+-  InputSameDT=on  SaturateOnIntegerOverflow=on  OutDataTypeStr=Inherit: Same as first input
  Sum3 : Sum  Inputs=+++  InputSameDT=on  SaturateOnIntegerOverflow=on  OutDataTypeStr=Inherit: Same as first input
  Sum4 : Sum  Inputs=+-  InputSameDT=on  SaturateOnIntegerOverflow=on  OutDataTypeStr=Inherit: Same as first input
  Sum5 : Sum  Inputs=+-+  InputSameDT=on  SaturateOnIntegerOverflow=on  OutDataTypeStr=Inherit: Same as first input
  Sum6 : Sum  Inputs=+++  InputSameDT=on  SaturateOnIntegerOverflow=on  OutDataTypeStr=Inherit: Same as first input
  gain1 : Gain  Gain=2  SaturateOnIntegerOverflow=on  OutDataTypeStr=Inherit: Same as input  ParamDataTypeStr=Inherit: Same as input
  gain2 : Gain  Gain=2*pi  SaturateOnIntegerOverflow=on  OutDataTypeStr=Inherit: Same as input  ParamDataTypeStr=Inherit: Same as input
  gain3 : Gain  Gain=2  SaturateOnIntegerOverflow=on  OutDataTypeStr=Inherit: Same as input  ParamDataTypeStr=Inherit: Same as input
  gain4 : Gain  Gain=4  SaturateOnIntegerOverflow=on  OutDataTypeStr=Inherit: Same as input  ParamDataTypeStr=Inherit: Same as input
  "x(n), x(n-1), x(n-2)" : Product  RndMeth=Zero
  y(n-1) : Product  RndMeth=Zero
  y(n-2) : Product  RndMeth=Zero
  Out : Outport  VectorParamsAs1DForOutWhenUnconnected=off
  wires:
  Product1/1 -> Out/1, Delay3/1, Delay2/1
  Sum2/1 -> Product1/1
  fc/1 -> gain2/1
  In/1 -> Delay1/1, Delay/1, Sum3/1
  gain2/1 -> Product3/1, Product2/2, Product2/1
  Constant/1 -> Product3/2, Product2/4, Product2/3
  Delay1/1 -> gain1/1
  gain1/1 -> Sum3/2
  Delay/1 -> Sum3/3
  Sum3/1 -> "x(n), x(n-1), x(n-2)"/1
  Product2/1 -> Sum5/1, Sum6/1, "x(n), x(n-1), x(n-2)"/2, gain3/1
  "x(n), x(n-1), x(n-2)"/1 -> Sum1/1
  Sum1/1 -> Sum2/1
  y(n-1)/1 -> Sum1/2
  Sum4/1 -> y(n-1)/1
  gain3/1 -> Sum4/1
  Constant1/1 -> Sum4/2
  Delay2/1 -> y(n-1)/2
  Product3/1 -> gain4/1
  Constant2/1 -> Sum5/3, Sum6/3
  Sum5/1 -> y(n-2)/1
  Delay3/1 -> y(n-2)/2
  y(n-2)/1 -> Sum2/2
  Sum6/1 -> Product1/2
  zeta/1 -> Product4/2
  gain4/1 -> Product4/1
  Product4/1 -> Sum6/2, Sum5/2

== system Katex_FullCar_R2017b_V03/DGIST/_Low_Level_Ctrl/Steering_Low_Level_Controller/Torque Mode/Steering Motor Control2/Lag compensator(zeta)/Dot1 ==
  note: Dot
  in : Inport
  Sum1 : Sum  Inputs=+-  InputSameDT=on  SaturateOnIntegerOverflow=on  OutDataTypeStr=Inherit: Same as first input
  Sum2 : Sum  Inputs=+-  InputSameDT=on  SaturateOnIntegerOverflow=on  OutDataTypeStr=Inherit: Same as first input
  d : UnitDelay  SampleTime=Ts
  d1 : UnitDelay  SampleTime=Ts
  gain : Gain  Gain=2/Ts  SaturateOnIntegerOverflow=on  OutDataTypeStr=Inherit: Same as input  ParamDataTypeStr=Inherit: Same as input
  out : Outport  VectorParamsAs1DForOutWhenUnconnected=off
  wires:
  Sum1/1 -> d1/1, out/1
  d1/1 -> Sum1/2
  Sum2/1 -> gain/1
  in/1 -> d/1, Sum2/1
  d/1 -> Sum2/2
  gain/1 -> Sum1/1

== system Katex_FullCar_R2017b_V03/DGIST/_Low_Level_Ctrl/Steering_Low_Level_Controller/Torque Mode/Steering Motor Control2/Lag compensator(zeta)/a//(s+p) ==
  note: y(n) = [(2-p*Ts)*y(n-1)+a*Ts(u(n)+u(n-1))]/(2+p*Ts)
  note: H(s) = a/(s+p)
  note: s = 2/Ts*(z-1)/(z+1)
  In : Inport
  a : Inport  Port=2
  p : Inport  Port=3
  Constant : Constant  Value=2  SampleTime=Ts
  Product1 : Product  Inputs=*/  RndMeth=Zero
  Product11 : Product  RndMeth=Zero
  Product3 : Product  RndMeth=Zero
  Sum1 : Sum  Inputs=-+  InputSameDT=on  SaturateOnIntegerOverflow=on  OutDataTypeStr=Inherit: Same as first input
  Sum2 : Sum  InputSameDT=on  SaturateOnIntegerOverflow=on  OutDataTypeStr=Inherit: Same as first input
  Sum3 : Sum  InputSameDT=on  SaturateOnIntegerOverflow=on  OutDataTypeStr=Inherit: Same as first input
  Sum4 : Sum  InputSameDT=on  SaturateOnIntegerOverflow=on  OutDataTypeStr=Inherit: Same as first input
  d : UnitDelay  SampleTime=Ts
  d1 : UnitDelay  SampleTime=Ts
  gain : Gain  Gain=Ts  SaturateOnIntegerOverflow=on  OutDataTypeStr=Inherit: Same as input  ParamDataTypeStr=Inherit: Same as input
  gain1 : Gain  Gain=Ts  SaturateOnIntegerOverflow=on  OutDataTypeStr=Inherit: Same as input  ParamDataTypeStr=Inherit: Same as input
  Out : Outport  VectorParamsAs1DForOutWhenUnconnected=off
  wires:
  In/1 -> Sum3/1, d1/1
  d1/1 -> Sum3/2
  Sum3/1 -> gain/1
  Product11/1 -> Sum2/2
  Sum1/1 -> Product11/1
  Constant/1 -> Sum1/2, Sum4/2
  p/1 -> gain1/1
  gain1/1 -> Sum1/1, Sum4/1
  d/1 -> Product11/2
  Sum2/1 -> Product1/1
  Sum4/1 -> Product1/2
  Product1/1 -> Out/1, d/1
  gain/1 -> Product3/1
  a/1 -> Product3/2
  Product3/1 -> Sum2/1

== system Katex_FullCar_R2017b_V03/DGIST/_Low_Level_Ctrl/Steering_Low_Level_Controller/Torque Mode/Steering Motor Control2/Poleplacement(PI)1/Integrator1 ==
  note: Integrator
  in : Inport
  "Off : 0 On : 1" : Inport  Port=2
  Divide : Product  Inputs=**
  Sum1 : Sum  InputSameDT=on  SaturateOnIntegerOverflow=on  OutDataTypeStr=Inherit: Same as first input
  Sum2 : Sum  InputSameDT=on  SaturateOnIntegerOverflow=on  OutDataTypeStr=Inherit: Same as first input
  d : UnitDelay  SampleTime=Ts
  d1 : UnitDelay  SampleTime=Ts
  gain : Gain  Gain=Ts/2  SaturateOnIntegerOverflow=on  OutDataTypeStr=Inherit: Same as input  ParamDataTypeStr=Inherit: Same as input
  out : Outport  VectorParamsAs1DForOutWhenUnconnected=off
  wires:
  gain/1 -> Sum2/1
  Sum1/1 -> gain/1
  d1/1 -> Sum1/2
  in/1 -> d1/1, Sum1/1
  Sum2/1 -> Divide/1, out/1
  d/1 -> Sum2/2
  Divide/1 -> d/1
  "Off : 0 On : 1"/1 -> Divide/2

== system Katex_FullCar_R2017b_V03/DGIST/_Low_Level_Ctrl/Steering_Low_Level_Controller/Torque Mode/Steering Motor Control2/Steering Ref Mode /If Action Subsystem ==
  In1 : Inport
  Action Port : ActionPort
  Out1 : Outport  VectorParamsAs1DForOutWhenUnconnected=off
  wires:
  In1/1 -> Out1/1

== system Katex_FullCar_R2017b_V03/DGIST/_Low_Level_Ctrl/Steering_Low_Level_Controller/Torque Mode/Steering Motor Control2/Steering Ref Mode /If Action Subsystem1 ==
  In1 : Inport
  Action Port : ActionPort
  Out1 : Outport  VectorParamsAs1DForOutWhenUnconnected=off
  wires:
  In1/1 -> Out1/1

== system Katex_FullCar_R2017b_V03/DGIST/_Low_Level_Ctrl/Steering_Low_Level_Controller/Torque Mode/Steering Motor Control2/Steering Ref Mode /If Action Subsystem2 ==
  In1 : Inport
  Action Port : ActionPort
  Out1 : Outport  VectorParamsAs1DForOutWhenUnconnected=off
  wires:
  In1/1 -> Out1/1

== system Katex_FullCar_R2017b_V03/DGIST/_Low_Level_Ctrl/Steering_Low_Level_Controller/Torque Mode/Steering Motor Control3/DOB(theta)/Dot ==
  note: Dot
  in : Inport
  Sum1 : Sum  Inputs=+-  InputSameDT=on  SaturateOnIntegerOverflow=on  OutDataTypeStr=Inherit: Same as first input
  Sum2 : Sum  Inputs=+-  InputSameDT=on  SaturateOnIntegerOverflow=on  OutDataTypeStr=Inherit: Same as first input
  d : UnitDelay  SampleTime=Ts
  d1 : UnitDelay  SampleTime=Ts
  gain : Gain  Gain=2/Ts  SaturateOnIntegerOverflow=on  OutDataTypeStr=Inherit: Same as input  ParamDataTypeStr=Inherit: Same as input
  out : Outport  VectorParamsAs1DForOutWhenUnconnected=off
  wires:
  Sum1/1 -> d1/1, out/1
  d1/1 -> Sum1/2
  Sum2/1 -> gain/1
  in/1 -> d/1, Sum2/1
  d/1 -> Sum2/2
  gain/1 -> Sum1/1

== system Katex_FullCar_R2017b_V03/DGIST/_Low_Level_Ctrl/Steering_Low_Level_Controller/Torque Mode/Steering Motor Control3/DOB(theta)/Dot1 ==
  note: Dot
  in : Inport
  Sum1 : Sum  Inputs=+-  InputSameDT=on  SaturateOnIntegerOverflow=on  OutDataTypeStr=Inherit: Same as first input
  Sum2 : Sum  Inputs=+-  InputSameDT=on  SaturateOnIntegerOverflow=on  OutDataTypeStr=Inherit: Same as first input
  d : UnitDelay  SampleTime=Ts
  d1 : UnitDelay  SampleTime=Ts
  gain : Gain  Gain=2/Ts  SaturateOnIntegerOverflow=on  OutDataTypeStr=Inherit: Same as input  ParamDataTypeStr=Inherit: Same as input
  out : Outport  VectorParamsAs1DForOutWhenUnconnected=off
  wires:
  Sum1/1 -> d1/1, out/1
  d1/1 -> Sum1/2
  Sum2/1 -> gain/1
  in/1 -> d/1, Sum2/1
  d/1 -> Sum2/2
  gain/1 -> Sum1/1

== system Katex_FullCar_R2017b_V03/DGIST/_Low_Level_Ctrl/Steering_Low_Level_Controller/Torque Mode/Steering Motor Control3/DOB(theta)/Dot2 ==
  note: Dot
  in : Inport
  Sum1 : Sum  Inputs=+-  InputSameDT=on  SaturateOnIntegerOverflow=on  OutDataTypeStr=Inherit: Same as first input
  Sum2 : Sum  Inputs=+-  InputSameDT=on  SaturateOnIntegerOverflow=on  OutDataTypeStr=Inherit: Same as first input
  d : UnitDelay  SampleTime=Ts
  d1 : UnitDelay  SampleTime=Ts
  gain : Gain  Gain=2/Ts  SaturateOnIntegerOverflow=on  OutDataTypeStr=Inherit: Same as input  ParamDataTypeStr=Inherit: Same as input
  out : Outport  VectorParamsAs1DForOutWhenUnconnected=off
  wires:
  Sum1/1 -> d1/1, out/1
  d1/1 -> Sum1/2
  Sum2/1 -> gain/1
  in/1 -> d/1, Sum2/1
  d/1 -> Sum2/2
  gain/1 -> Sum1/1

== system Katex_FullCar_R2017b_V03/DGIST/_Low_Level_Ctrl/Steering_Low_Level_Controller/Torque Mode/Steering Motor Control3/DOB(theta)/Second order LPF ==
  note: y(n) = [Ts^2*w^2*{x(n)+2*x(n-1)+x(n-2)}-(2*w^2*Ts^2-8)*y(n-1)-(4+w^2*Ts^2+2*zeta*Ts*w)*y(n-2)]
      | /(4+w^2*Ts^2+2*zeta*Ts*w)
  note: H(s) = w^2/(s^2+2*zeta*w*s+w^2)
  note: s = 2/Ts*(z-1)/(z+1)
  In : Inport
  fc : Inport  Port=2
  zeta : Inport  Port=3
  Constant : Constant  Value=Ts  SampleTime=Ts
  Constant1 : Constant  Value=8  SampleTime=Ts
  Constant2 : Constant  Value=4  SampleTime=Ts
  Delay : Delay  InitialCondition=0  SampleTime=Ts
  Delay1 : Delay  DelayLength=1  InitialCondition=0  SampleTime=Ts
  Delay2 : Delay  DelayLength=1  InitialCondition=0  SampleTime=Ts
  Delay3 : Delay  InitialCondition=0  SampleTime=Ts
  Product1 : Product  Inputs=*/  RndMeth=Zero
  Product2 : Product  Inputs=4  RndMeth=Zero
  Product3 : Product  RndMeth=Zero
  Product4 : Product  RndMeth=Zero
  Sum1 : Sum  Inputs=+-  InputSameDT=on  SaturateOnIntegerOverflow=on  OutDataTypeStr=Inherit: Same as first input
  Sum2 : Sum  Inputs=+-  InputSameDT=on  SaturateOnIntegerOverflow=on  OutDataTypeStr=Inherit: Same as first input
  Sum3 : Sum  Inputs=+++  InputSameDT=on  SaturateOnIntegerOverflow=on  OutDataTypeStr=Inherit: Same as first input
  Sum4 : Sum  Inputs=+-  InputSameDT=on  SaturateOnIntegerOverflow=on  OutDataTypeStr=Inherit: Same as first input
  Sum5 : Sum  Inputs=+-+  InputSameDT=on  SaturateOnIntegerOverflow=on  OutDataTypeStr=Inherit: Same as first input
  Sum6 : Sum  Inputs=+++  InputSameDT=on  SaturateOnIntegerOverflow=on  OutDataTypeStr=Inherit: Same as first input
  gain1 : Gain  Gain=2  SaturateOnIntegerOverflow=on  OutDataTypeStr=Inherit: Same as input  ParamDataTypeStr=Inherit: Same as input
  gain2 : Gain  Gain=2*pi  SaturateOnIntegerOverflow=on  OutDataTypeStr=Inherit: Same as input  ParamDataTypeStr=Inherit: Same as input
  gain3 : Gain  Gain=2  SaturateOnIntegerOverflow=on  OutDataTypeStr=Inherit: Same as input  ParamDataTypeStr=Inherit: Same as input
  gain4 : Gain  Gain=4  SaturateOnIntegerOverflow=on  OutDataTypeStr=Inherit: Same as input  ParamDataTypeStr=Inherit: Same as input
  "x(n), x(n-1), x(n-2)" : Product  RndMeth=Zero
  y(n-1) : Product  RndMeth=Zero
  y(n-2) : Product  RndMeth=Zero
  Dist_hat : Outport  VectorParamsAs1DForOutWhenUnconnected=off
  wires:
  Product1/1 -> Dist_hat/1, Delay3/1, Delay2/1
  Sum2/1 -> Product1/1
  fc/1 -> gain2/1
  In/1 -> Delay1/1, Delay/1, Sum3/1
  gain2/1 -> Product3/1, Product2/2, Product2/1
  Constant/1 -> Product3/2, Product2/4, Product2/3
  Delay1/1 -> gain1/1
  gain1/1 -> Sum3/2
  Delay/1 -> Sum3/3
  Sum3/1 -> "x(n), x(n-1), x(n-2)"/1
  Product2/1 -> Sum5/1, Sum6/1, "x(n), x(n-1), x(n-2)"/2, gain3/1
  "x(n), x(n-1), x(n-2)"/1 -> Sum1/1
  Sum1/1 -> Sum2/1
  y(n-1)/1 -> Sum1/2
  Sum4/1 -> y(n-1)/1
  gain3/1 -> Sum4/1
  Constant1/1 -> Sum4/2
  Delay2/1 -> y(n-1)/2
  Product3/1 -> gain4/1
  Constant2/1 -> Sum5/3, Sum6/3
  Sum5/1 -> y(n-2)/1
  Delay3/1 -> y(n-2)/2
  y(n-2)/1 -> Sum2/2
  Sum6/1 -> Product1/2
  zeta/1 -> Product4/2
  gain4/1 -> Product4/1
  Product4/1 -> Sum6/2, Sum5/2

== system Katex_FullCar_R2017b_V03/DGIST/_Low_Level_Ctrl/Steering_Low_Level_Controller/Torque Mode/Steering Motor Control3/Feedforward(theta)/Dot ==
  note: Dot
  in : Inport
  Sum1 : Sum  Inputs=+-  InputSameDT=on  SaturateOnIntegerOverflow=on  OutDataTypeStr=Inherit: Same as first input
  Sum2 : Sum  Inputs=+-  InputSameDT=on  SaturateOnIntegerOverflow=on  OutDataTypeStr=Inherit: Same as first input
  d : UnitDelay  SampleTime=Ts
  d1 : UnitDelay  SampleTime=Ts
  gain : Gain  Gain=2/Ts  SaturateOnIntegerOverflow=on  OutDataTypeStr=Inherit: Same as input  ParamDataTypeStr=Inherit: Same as input
  out : Outport  VectorParamsAs1DForOutWhenUnconnected=off
  wires:
  Sum1/1 -> d1/1, out/1
  d1/1 -> Sum1/2
  Sum2/1 -> gain/1
  in/1 -> d/1, Sum2/1
  d/1 -> Sum2/2
  gain/1 -> Sum1/1

== system Katex_FullCar_R2017b_V03/DGIST/_Low_Level_Ctrl/Steering_Low_Level_Controller/Torque Mode/Steering Motor Control3/Feedforward(theta)/Dot1 ==
  note: Dot
  in : Inport
  Sum1 : Sum  Inputs=+-  InputSameDT=on  SaturateOnIntegerOverflow=on  OutDataTypeStr=Inherit: Same as first input
  Sum2 : Sum  Inputs=+-  InputSameDT=on  SaturateOnIntegerOverflow=on  OutDataTypeStr=Inherit: Same as first input
  d : UnitDelay  SampleTime=Ts
  d1 : UnitDelay  SampleTime=Ts
  gain : Gain  Gain=2/Ts  SaturateOnIntegerOverflow=on  OutDataTypeStr=Inherit: Same as input  ParamDataTypeStr=Inherit: Same as input
  out : Outport  VectorParamsAs1DForOutWhenUnconnected=off
  wires:
  Sum1/1 -> d1/1, out/1
  d1/1 -> Sum1/2
  Sum2/1 -> gain/1
  in/1 -> d/1, Sum2/1
  d/1 -> Sum2/2
  gain/1 -> Sum1/1

== system Katex_FullCar_R2017b_V03/DGIST/_Low_Level_Ctrl/Steering_Low_Level_Controller/Torque Mode/Steering Motor Control3/Feedforward(theta)/Dot2 ==
  note: Dot
  in : Inport
  Sum1 : Sum  Inputs=+-  InputSameDT=on  SaturateOnIntegerOverflow=on  OutDataTypeStr=Inherit: Same as first input
  Sum2 : Sum  Inputs=+-  InputSameDT=on  SaturateOnIntegerOverflow=on  OutDataTypeStr=Inherit: Same as first input
  d : UnitDelay  SampleTime=Ts
  d1 : UnitDelay  SampleTime=Ts
  gain : Gain  Gain=2/Ts  SaturateOnIntegerOverflow=on  OutDataTypeStr=Inherit: Same as input  ParamDataTypeStr=Inherit: Same as input
  out : Outport  VectorParamsAs1DForOutWhenUnconnected=off
  wires:
  Sum1/1 -> d1/1, out/1
  d1/1 -> Sum1/2
  Sum2/1 -> gain/1
  in/1 -> d/1, Sum2/1
  d/1 -> Sum2/2
  gain/1 -> Sum1/1

== system Katex_FullCar_R2017b_V03/DGIST/_Low_Level_Ctrl/Steering_Low_Level_Controller/Torque Mode/Steering Motor Control3/Feedforward(theta)/Second order LPF ==
  note: y(n) = [Ts^2*w^2*{x(n)+2*x(n-1)+x(n-2)}-(2*w^2*Ts^2-8)*y(n-1)-(4+w^2*Ts^2+2*zeta*Ts*w)*y(n-2)]
      | /(4+w^2*Ts^2+2*zeta*Ts*w)
  note: H(s) = w^2/(s^2+2*zeta*w*s+w^2)
  note: s = 2/Ts*(z-1)/(z+1)
  In : Inport
  fc : Inport  Port=2
  zeta : Inport  Port=3
  Constant : Constant  Value=Ts  SampleTime=Ts
  Constant1 : Constant  Value=8  SampleTime=Ts
  Constant2 : Constant  Value=4  SampleTime=Ts
  Delay : Delay  InitialCondition=0  SampleTime=Ts
  Delay1 : Delay  DelayLength=1  InitialCondition=0  SampleTime=Ts
  Delay2 : Delay  DelayLength=1  InitialCondition=0  SampleTime=Ts
  Delay3 : Delay  InitialCondition=0  SampleTime=Ts
  Product1 : Product  Inputs=*/  RndMeth=Zero
  Product2 : Product  Inputs=4  RndMeth=Zero
  Product3 : Product  RndMeth=Zero
  Product4 : Product  RndMeth=Zero
  Sum1 : Sum  Inputs=+-  InputSameDT=on  SaturateOnIntegerOverflow=on  OutDataTypeStr=Inherit: Same as first input
  Sum2 : Sum  Inputs=+-  InputSameDT=on  SaturateOnIntegerOverflow=on  OutDataTypeStr=Inherit: Same as first input
  Sum3 : Sum  Inputs=+++  InputSameDT=on  SaturateOnIntegerOverflow=on  OutDataTypeStr=Inherit: Same as first input
  Sum4 : Sum  Inputs=+-  InputSameDT=on  SaturateOnIntegerOverflow=on  OutDataTypeStr=Inherit: Same as first input
  Sum5 : Sum  Inputs=+-+  InputSameDT=on  SaturateOnIntegerOverflow=on  OutDataTypeStr=Inherit: Same as first input
  Sum6 : Sum  Inputs=+++  InputSameDT=on  SaturateOnIntegerOverflow=on  OutDataTypeStr=Inherit: Same as first input
  gain1 : Gain  Gain=2  SaturateOnIntegerOverflow=on  OutDataTypeStr=Inherit: Same as input  ParamDataTypeStr=Inherit: Same as input
  gain2 : Gain  Gain=2*pi  SaturateOnIntegerOverflow=on  OutDataTypeStr=Inherit: Same as input  ParamDataTypeStr=Inherit: Same as input
  gain3 : Gain  Gain=2  SaturateOnIntegerOverflow=on  OutDataTypeStr=Inherit: Same as input  ParamDataTypeStr=Inherit: Same as input
  gain4 : Gain  Gain=4  SaturateOnIntegerOverflow=on  OutDataTypeStr=Inherit: Same as input  ParamDataTypeStr=Inherit: Same as input
  "x(n), x(n-1), x(n-2)" : Product  RndMeth=Zero
  y(n-1) : Product  RndMeth=Zero
  y(n-2) : Product  RndMeth=Zero
  Out : Outport  VectorParamsAs1DForOutWhenUnconnected=off
  wires:
  Product1/1 -> Out/1, Delay3/1, Delay2/1
  Sum2/1 -> Product1/1
  fc/1 -> gain2/1
  In/1 -> Delay1/1, Delay/1, Sum3/1
  gain2/1 -> Product3/1, Product2/2, Product2/1
  Constant/1 -> Product3/2, Product2/4, Product2/3
  Delay1/1 -> gain1/1
  gain1/1 -> Sum3/2
  Delay/1 -> Sum3/3
  Sum3/1 -> "x(n), x(n-1), x(n-2)"/1
  Product2/1 -> Sum5/1, Sum6/1, "x(n), x(n-1), x(n-2)"/2, gain3/1
  "x(n), x(n-1), x(n-2)"/1 -> Sum1/1
  Sum1/1 -> Sum2/1
  y(n-1)/1 -> Sum1/2
  Sum4/1 -> y(n-1)/1
  gain3/1 -> Sum4/1
  Constant1/1 -> Sum4/2
  Delay2/1 -> y(n-1)/2
  Product3/1 -> gain4/1
  Constant2/1 -> Sum5/3, Sum6/3
  Sum5/1 -> y(n-2)/1
  Delay3/1 -> y(n-2)/2
  y(n-2)/1 -> Sum2/2
  Sum6/1 -> Product1/2
  zeta/1 -> Product4/2
  gain4/1 -> Product4/1
  Product4/1 -> Sum6/2, Sum5/2
